simulink model "simulink_for_task5"  (R2023a)
settings: Solver=VariableStepAuto  StartTime=0.0  StopTime=10.0  RelTol=1e-3
values from neighbouring files (symbols this model uses):
  CA0 = 0.5    [param_consts.m]
  CAf = 1.0    (= 1)    [param_consts.m]
  Cp = 0.239    [param_consts.m]
  dHr = -5e4    (= -50000)    [param_consts.m]
  ER = 8750    [param_consts.m]
  k0 = 5e10    (= 50000000000)    [param_consts.m]
  q = 100    [param_consts.m]
  rho = 1000    [param_consts.m]
  T0 = 305    [param_consts.m]
  Tc = 270    [param_consts.m]
  Tf = 350    [param_consts.m]
  UA = 5e4    (= 50000)    [param_consts.m]
  V = 100    [param_consts.m]
settings Model: Creator=xiong  LastModifiedBy=xiong

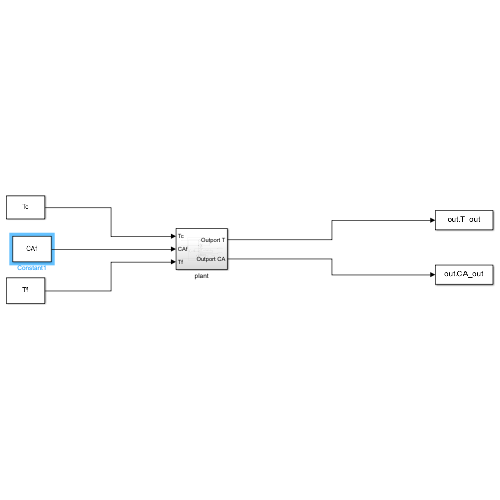
[thumbnail: Simulink's stored preview of the top-level diagram]
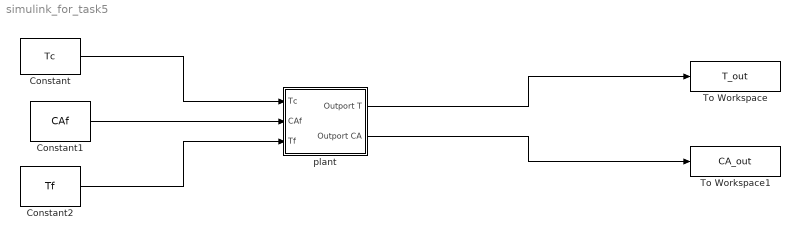
== system simulink_for_task5 ==
  Constant : Constant  Value=Tc
  Constant1 : Constant  Value=CAf
  Constant2 : Constant  Value=Tf
  To Workspace : ToWorkspace  VariableName=T_out  SaveFormat=Structure With Time  SampleTime=-1
  To Workspace1 : ToWorkspace  VariableName=CA_out  SaveFormat=Structure With Time  SampleTime=-1
  plant : Subsystem
  wires:
  plant/1(Outport T) -> To Workspace/1
  plant/2(Outport CA) -> To Workspace1/1
  Constant/1 -> plant/1(Tc)
  Constant1/1 -> plant/2(CAf)
  Constant2/1 -> plant/3(Tf)

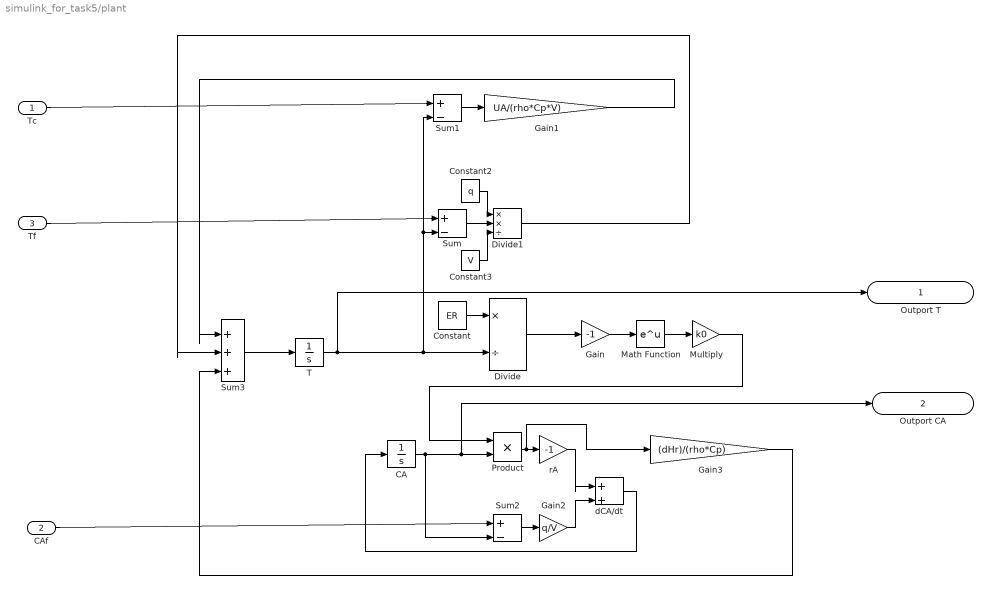
== system simulink_for_task5/plant ==
  Tc : Inport
  CAf : Inport  Port=2
  Tf : Inport  Port=3
  CA : Integrator  InitialCondition=CA0
  Constant : Constant  Value=ER
  Constant2 : Constant  Value=q
  Constant3 : Constant  Value=V
  Divide : Product  Inputs=*/
  Divide1 : Product  Inputs=**/
  Gain : Gain  Gain=-1
  Gain1 : Gain  Gain=UA/(rho*Cp*V)
  Gain2 : Gain  Gain=q/V
  Gain3 : Gain  Gain=(dHr)/(rho*Cp)
  Math Function : Math
  Multiply : Gain  Gain=k0
  Product : Product
  Sum : Sum  Inputs=|+-
  Sum1 : Sum  Inputs=|+-
  Sum2 : Sum  Inputs=|+-
  Sum3 : Sum  Inputs=|+++
  T : Integrator  Tag=T  InitialCondition=T0  ContinuousStateAttributes='T'
  dCA/dt : Sum  Inputs=|++
  rA : Gain  Gain=-1
  Outport T : Outport
  Outport CA : Outport  Port=2
  wires:
  Multiply/1 -> Product/1
  Sum/1 -> Divide1/2
  T/1 -> Outport T/1, Sum1/2, Sum/2, Divide/2
  Gain/1 -> Math Function/1
  Divide1/1 -> Sum3/2
  Product/1 -> Gain3/1, rA/1
  Gain1/1 -> Sum3/1
  CA/1 -> Outport CA/1, Product/2, Sum2/2
  CAf/1 -> Sum2/1
  Divide/1 -> Gain/1
  Constant/1 -> Divide/1
  rA/1 -> dCA/dt/1
  Tc/1 -> Sum1/1
  Sum2/1 -> Gain2/1
  Constant3/1 -> Divide1/3
  dCA/dt/1 -> CA/1
  Tf/1 -> Sum/1
  Math Function/1 -> Multiply/1
  Constant2/1 -> Divide1/1
  Sum3/1 -> T/1
  Gain3/1 -> Sum3/3
  Gain2/1 -> dCA/dt/2
  Sum1/1 -> Gain1/1
